simulink model "ctrlAllocMatrix_th"  (R2018b)
settings: Solver=VariableStepAuto  StartTime=0.0  StopTime=0  RelTol=1e-3
values from neighbouring files (symbols this model uses):
  angVelBdy = [0 0 0]*pi/180    [ctrlAllocMatrix_ts.m]
  momDesBdy = -1e4*[1 1 1]    [ctrlAllocMatrix_ts.m]
  velCMBdy = 2*[-2 0 -0.1]    [ctrlAllocMatrix_ts.m]
  velWndBdy = [0 0 0]    [ctrlAllocMatrix_ts.m]
undefined symbols (not defined in the file or in its folder): vhcl
libraries: ctrlAllocMatrix_cl x1, fluidDynamicSurface_cl x1
settings Model: Creator=mcobb  LastModifiedBy=mcobb

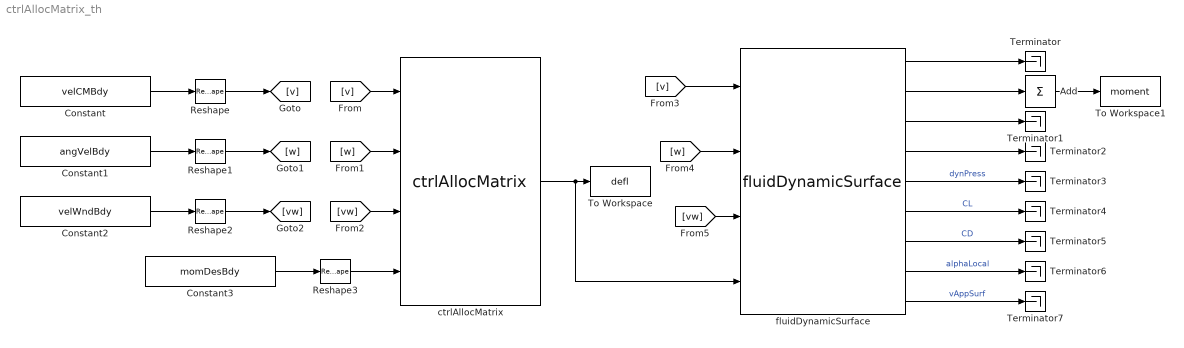
== system ctrlAllocMatrix_th ==
  Add : Sum  Inputs=1  CollapseMode=Specified dimension  CollapseDim=2
  Constant : Constant  Value=velCMBdy
  Constant1 : Constant  Value=angVelBdy
  Constant2 : Constant  Value=velWndBdy
  Constant3 : Constant  Value=momDesBdy
  Reshape{,1..3} (4 alike) : Reshape  OutputDimensionality=Column vector (2-D)
  Terminator{,1..7} (8 alike) : Terminator
  To Workspace : ToWorkspace  VariableName=defl  SaveFormat=Timeseries  SampleTime=-1
  To Workspace1 : ToWorkspace  VariableName=moment  SaveFormat=Timeseries  SampleTime=-1
  ctrlAllocMatrix : ctrlAllocMatrix_cl/ctrlAllocMatrix  aeroStruct=vhcl.struct('OCT.aeroSurf')  fluidDensity=1000  ctrlUpMax=30  ctrlDnMax=-30
  fluidDynamicSurface : fluidDynamicSurface_cl/fluidDynamicSurface  aeroStruct=vhcl.struct('OCT.aeroSurf')  fluidDensity=1000
  wires:
  Constant/1 -> Reshape/1
  Constant1/1 -> Reshape1/1
  Constant2/1 -> Reshape2/1
  Constant3/1 -> Reshape3/1
  Reshape3/1 -> ctrlAllocMatrix/4
  ctrlAllocMatrix/1 -> fluidDynamicSurface/4, To Workspace/1
  Reshape/1 -> [v]
  [v] -> ctrlAllocMatrix/1
  [w] -> ctrlAllocMatrix/2
  Reshape1/1 -> [w]
  Reshape2/1 -> [vw]
  [vw] -> ctrlAllocMatrix/3
  [v] -> fluidDynamicSurface/1
  [w] -> fluidDynamicSurface/2
  [vw] -> fluidDynamicSurface/3
  fluidDynamicSurface/1 -> Terminator/1
  fluidDynamicSurface/2 -> Add/1
  fluidDynamicSurface/3 -> Terminator1/1
  fluidDynamicSurface/4 -> Terminator2/1
  fluidDynamicSurface/5 -> Terminator3/1  "dynPress"
  fluidDynamicSurface/6 -> Terminator4/1  "CL"
  fluidDynamicSurface/7 -> Terminator5/1  "CD"
  fluidDynamicSurface/8 -> Terminator6/1  "alphaLocal"
  fluidDynamicSurface/9 -> Terminator7/1  "vAppSurf"
  Add/1 -> To Workspace1/1
